simulink model "simulator_prototype_v2"  (R2021b)
settings: Solver=ode15s  StartTime=0.0  StopTime=200  FixedStep=0.01  RelTol=1e-3
(part 1 of 12)
settings Model: Creator=anlun  LastModifiedBy=anlun

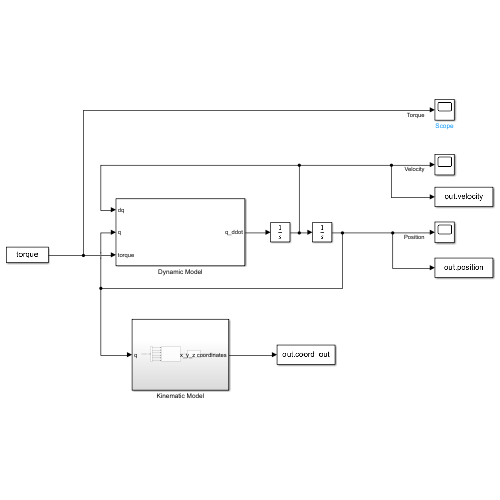
[thumbnail: Simulink's stored preview of the top-level diagram]
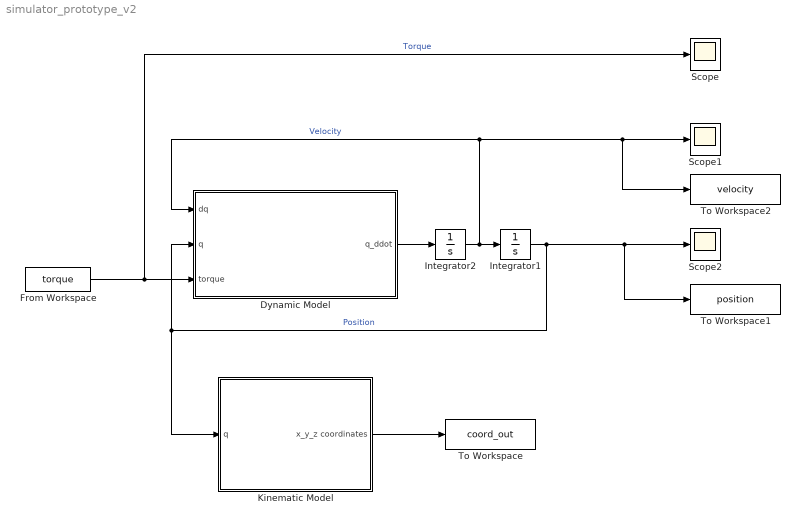
== system simulator_prototype_v2 ==
  Dynamic Model : Subsystem
  From Workspace : FromWorkspace  VariableName=torque
  Integrator1 : Integrator
  Integrator2 : Integrator
  Kinematic Model : Subsystem
  Scope : Scope
  Scope1 : Scope
  Scope2 : Scope
  To Workspace : ToWorkspace  VariableName=coord_out  SampleTime=-1
  To Workspace1 : ToWorkspace  VariableName=position  SampleTime=-1
  To Workspace2 : ToWorkspace  VariableName=velocity  SampleTime=-1
  wires:
  Integrator2/1 -> Integrator1/1, To Workspace2/1, Scope1/1, Dynamic Model/1(dq)  "Velocity"
  Integrator1/1 -> To Workspace1/1, Scope2/1, Kinematic Model/1(q), Dynamic Model/2(q)  "Position"
  From Workspace/1 -> Scope/1, Dynamic Model/3(torque)  "Torque"
  Dynamic Model/1(q_ddot) -> Integrator2/1
  Kinematic Model/1(x_y_z coordinates) -> To Workspace/1

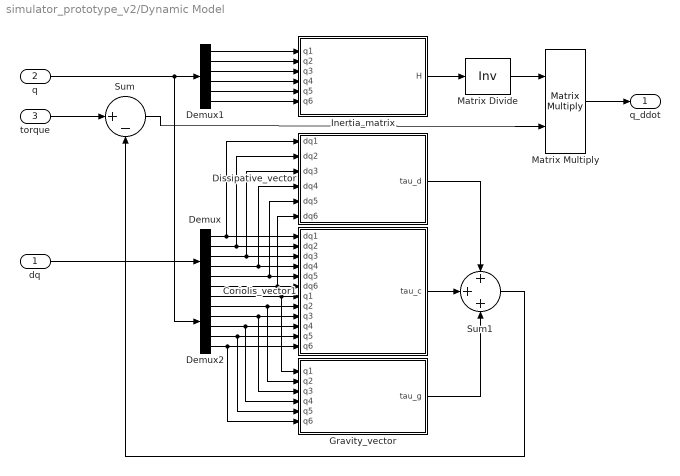
== system simulator_prototype_v2/Dynamic Model ==
  dq : Inport
  q : Inport  Port=2
  torque : Inport  Port=3
  Coriolis_vector1 : MATLAB Function  TreatAsAtomicUnit=on
  Demux : Demux  Outputs=6
  Demux1 : Demux  Outputs=6
  Demux2 : Demux  Outputs=6
  Dissipative_vector : MATLAB Function  TreatAsAtomicUnit=on
  Gravity_vector : MATLAB Function  TreatAsAtomicUnit=on
  Inertia_matrix : MATLAB Function  TreatAsAtomicUnit=on
  Matrix Divide : Product  Inputs=/  Multiplication=Matrix(*)
  Matrix Multiply : Product  Multiplication=Matrix(*)
  Sum : Sum  Inputs=|+-
  Sum1 : Sum  Inputs=+++
  q_ddot : Outport
  wires:
  torque/1 -> Sum/1
  Inertia_matrix/1(H) -> Matrix Divide/1
  Sum/1 -> Matrix Multiply/2
  Sum1/1 -> Sum/2
  Matrix Divide/1 -> Matrix Multiply/1
  Matrix Multiply/1 -> q_ddot/1
  dq/1 -> Demux/1
  Demux/1 -> Coriolis_vector1/1(dq1), Dissipative_vector/1(dq1)
  Demux/2 -> Coriolis_vector1/2(dq2), Dissipative_vector/2(dq2)
  Demux/3 -> Coriolis_vector1/3(dq3), Dissipative_vector/3(dq3)
  Demux/4 -> Coriolis_vector1/4(dq4), Dissipative_vector/4(dq4)
  Demux/5 -> Coriolis_vector1/5(dq5), Dissipative_vector/5(dq5)
  Demux/6 -> Dissipative_vector/6(dq6), Coriolis_vector1/6(dq6)
  Demux2/1 -> Gravity_vector/1(q1), Coriolis_vector1/7(q1)
  Demux2/2 -> Coriolis_vector1/8(q2), Gravity_vector/2(q2)
  Demux2/3 -> Coriolis_vector1/9(q3), Gravity_vector/3(q3)
  Demux2/4 -> Coriolis_vector1/10(q4), Gravity_vector/4(q4)
  Demux2/5 -> Coriolis_vector1/11(q5), Gravity_vector/5(q5)
  Demux2/6 -> Coriolis_vector1/12(q6), Gravity_vector/6(q6)
  q/1 -> Demux2/1, Demux1/1
  Coriolis_vector1/1(tau_c) -> Sum1/2
  Dissipative_vector/1(tau_d) -> Sum1/1
  Gravity_vector/1(tau_g) -> Sum1/3
  Demux1/1 -> Inertia_matrix/1(q1)
  Demux1/2 -> Inertia_matrix/2(q2)
  Demux1/3 -> Inertia_matrix/3(q3)
  Demux1/4 -> Inertia_matrix/4(q4)
  Demux1/5 -> Inertia_matrix/5(q5)
  Demux1/6 -> Inertia_matrix/6(q6)

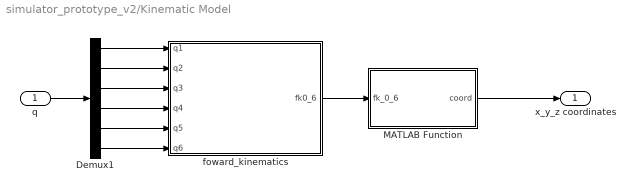
== system simulator_prototype_v2/Kinematic Model ==
  q : Inport
  Demux1 : Demux  Outputs=6
  MATLAB Function : MATLAB Function  TreatAsAtomicUnit=on
  foward_kinematics : MATLAB Function  TreatAsAtomicUnit=on
  x_y_z coordinates : Outport
  wires:
  q/1 -> Demux1/1
  Demux1/1 -> foward_kinematics/1(q1)
  Demux1/6 -> foward_kinematics/6(q6)
  Demux1/5 -> foward_kinematics/5(q5)
  Demux1/4 -> foward_kinematics/4(q4)
  Demux1/3 -> foward_kinematics/3(q3)
  Demux1/2 -> foward_kinematics/2(q2)
  foward_kinematics/1(fk0_6) -> MATLAB Function/1(fk_0_6)
  MATLAB Function/1(coord) -> x_y_z coordinates/1
